simulink model "salpChain1"  (Simulink 7.8)
settings: Solver=ode15s  StartTime=0.0  StopTime=400  RelTol=1e-3
values from neighbouring files (symbols this model uses):
  evenTorque = [0 0 0]    [15RunsSmallEtta.mat]    (also in 1To10withTorque.mat = [0 0 0.2]; 1To20Nodes.mat; 1To30HeadToTail.mat; 1To35FullFlip.mat)
  N = size(INPUT,1)    [SpinCalc.m]
  oddTorque = [0 0 0]    [15RunsSmallEtta.mat]    (also in 1To10withTorque.mat = [0 0 0.2]; 1To20Nodes.mat; 1To30HeadToTail.mat; 1To35FullFlip.mat)
  sInertia = [0.0008  0  0; 0  0.0008  0; 0  0  0.0004]    [15RunsSmallEtta.mat]    (also in 1To10withTorque.mat; 1To20Nodes.mat; 1To30HeadToTail.mat; 1To35FullFlip.mat)
  sMass = 0.04    [15RunsSmallEtta.mat]    (also in 1To10withTorque.mat; 1To20Nodes.mat; 1To30HeadToTail.mat; 1To35FullFlip.mat)
  uAmplitudeEven = [-1.03766578533 1.19688881264 1.2209450799]    [15RunsSmallEtta.mat]    (also in 1To10withTorque.mat = [-0.2 0 2]; 1To20Nodes.mat = [-0.2 0 2]; 1To30HeadToTail.mat = [-0.2 0 2]; 1To35FullFlip.mat = [-0.2 0.2 2])
libraries: mblibv1 x14
settings Model: Creator=benjJohnson  LastModifiedBy=benjJohnson

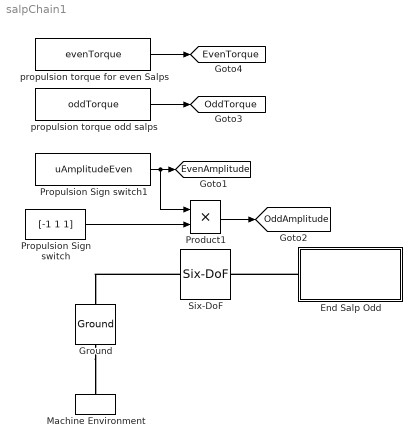
== system salpChain1 ==
  End Salp Odd : Subsystem
  Ground : mblibv1/Bodies/Ground  UpdateFromCAD=off  LeftPortType=env  RightPortType=workingframe  PhysicalDomain=Mechanical  DialogClass=GroundBlock  CoordPosition=[0 0 0]  CoordPositionUnits=m  StateVectorMgrId=-1  MachineId=[0 0]  ShowEnvPort=on
  Machine Environment : mblibv1/Bodies/Machine Environment  PortType=env  PhysicalDomain=Mechanical  DialogTemplateClass=MECH.MachineEnvironment  SyncWhenCopied=off  Gravity=[0 0 0]  GravityUnits=m/s^2  GravityAsSignal=off  Dimensionality=Auto-detect  AnalysisType=Forward dynamics  LinearAssemblyTolerance=1e-3  LinearAssemblyToleranceUnits=m  AngularAssemblyTolerance=1e-3  AngularAssemblyToleranceUnits=rad  ConstraintSolverType=Stabilizing  ConstraintRelTolerance=1e-4  ConstraintAbsTolerance=1e-4  UseRobustSingularityHandling=off  RedundancyAnalysisToleranceType=Automatically select tolerance  RedundancyAnalysisTolerance=1e-14  StatePerturbationType=Fixed  PerturbationSize=1e-5  VisualizeMachine=on  BodyVisualizationType=Use model default body geometries  BodyColorSelMode=Use model default  DefaultBodyColor=[1 0 0]
  Product1 : Product  RndMeth=Zero
  Propulsion Sign switch : Constant  Value=[-1 1 1]  VectorParams1D=off
  Propulsion Sign switch1 : Constant  Value=uAmplitudeEven  VectorParams1D=off
  Six-DoF : mblibv1/Joints/Six-DoF  LConnTagsString=__newl0  RConnTagsString=__newr0  UpdateFromCAD=off  NumSAPorts=0  CutJoint=off  MarkAsCut=off  Primitives=prismatic_prismatic  PrimitiveProps=P1$World$[1 0 0]$prismatic#P2$World$[0 1 0]$prismatic#P3$World$[0 0 1]$prismatic#S$World$[0 0 0]$spherical  DialogClass=JointBlock  P1Axis=[1 0 0]  P2Axis=[0 1 0]  P3Axis=[0 0 1]  SAxis=[0 0 0]
  propulsion torque for even Salps : Constant  Value=evenTorque  VectorParams1D=off
  propulsion torque odd salps : Constant  Value=oddTorque  VectorParams1D=off
  tag scope: EvenAmplitude=global, EvenTorque=global, OddAmplitude=global, OddTorque=global
  wires:
  Propulsion Sign switch/1 -> Product1/2
  Product1/1 -> [OddAmplitude]
  Propulsion Sign switch1/1 -> [EvenAmplitude], Product1/1
  propulsion torque for even Salps/1 -> [EvenTorque]
  propulsion torque odd salps/1 -> [OddTorque]
  connections:
  Six-DoF/LConn1 -- Ground/RConn1
  Ground/LConn1 -- Machine Environment/RConn1
  End Salp Odd/LConn1 -- Six-DoF/RConn1

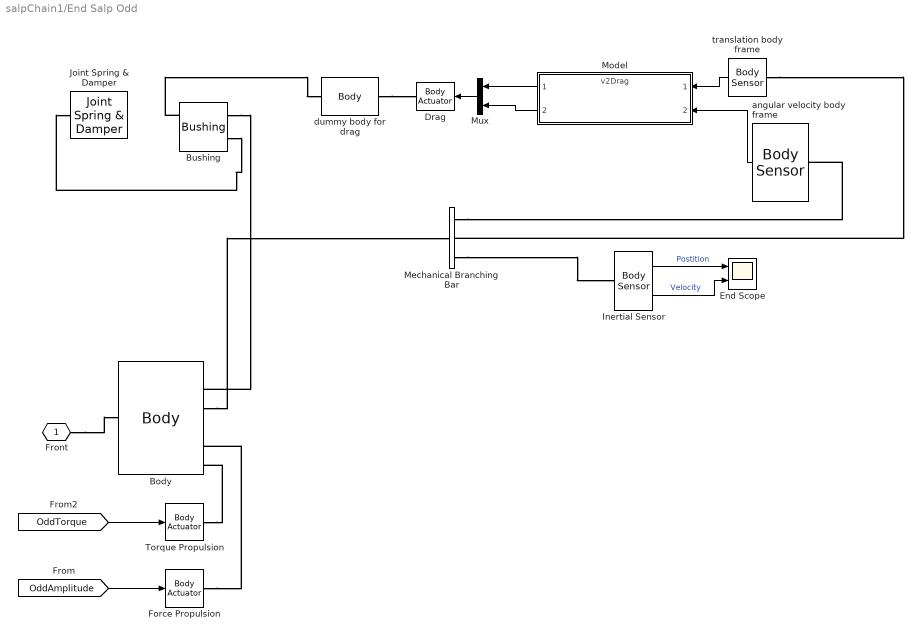
== system salpChain1/End Salp Odd ==
  Body : mblibv1/Bodies/Body  LConnTagsString=CS1  RConnTagsString=CG|CS5|CS4|CS2|CS3|CS6  UpdateFromCAD=off  DialogClass=MechanicalBodyBlock  Mass=sMass  MassUnits=kg  InertiaUnits=kg*m^2  Inertia=sInertia  Shape=Cylinder  ShapeDims=[1 1]  ShapeUnits=m  ShapeUse=false  Density=1  DensityUnits=kg/m^3  DensityUse=false  GraphicsMode=EQELLIPSE  BodyColorSelMode=COLORPALETTE  BodyColor=[0.16471 0.38431 0.27451]  AttachedToCS=CG  CG=Right$CG$frontConnect$CS1$CS1$m$[0 0 0]$Euler X-Y-Z$deg$CS1$true$none  WorkingFrames=Right$CS5$COPPosition$CG$CG$m$[0 0 0]$Euler X-Y-Z$deg$CS1$true$none#Right$CS4$[0 0 0]$CG$CG$m$[0 0 0]$Euler X-Y-Z$deg$CS1$true$none#Left$CS1$[0 0 0]$Adjoining$Adjoining$m$connectR$Euler X-Y-Z$deg$Adjoining$true$none#Right$CS2$backConnect$CG$CG$m$[0 0 0]$Euler X-Y-Z$deg$CS1$true$none#Right$CS3$propulsionPosition$CG$CG$m$[0 0 0]$Euler X-Y-Z$deg$CS1$true$none#Right$CS6$propulsionPosition$CG$CG$m$[0 0 0]$Euler X-Y-Z$deg$CS1$true$none  CGPos=frontConnect  CGRot=[0 0 0]  CS0Pos=[]  CS0Rot=[]  CS1Pos=[0 0 0]  CS1Rot=connectR  CS2Pos=backConnect  CS2Rot=[0 0 0]  CS3Pos=propulsionPosition  CS3Rot=[0 0 0]  CS4Pos=[0 0 0]  CS4Rot=[0 0 0]  CS5Pos=COPPosition  CS5Rot=[0 0 0]  CS6Pos=propulsionPosition  CS6Rot=[0 0 0]  CS7Pos=[]  CS7Rot=[]  CS8Pos=[]  CS8Rot=[]  CS9Pos=[]  CS9Rot=[]  CS10Pos=[]  CS10Rot=[]  CS11Pos=[]  CS11Rot=[]  CS12Pos=[]  CS12Rot=[]  CS13Pos=[]  CS13Rot=[]  CS14Pos=[]  CS14Rot=[]  CS15Pos=[]  CS15Rot=[]  CS16Pos=[]  CS16Rot=[]  CS17Pos=[]  CS17Rot=[]  CS18Pos=[]  CS18Rot=[]  CS19Pos=[]  CS19Rot=[]  CS20Pos=[]  CS20Rot=[]
  Bushing : mblibv1/Joints/Bushing  LConnTagsString=__newl0|SA1  RConnTagsString=__newr0|SA1  UpdateFromCAD=off  NumSAPorts=2  CutJoint=off  MarkAsCut=off  Primitives=prismatic_prismatic_prismatic  PrimitiveProps=P1$Follower$[1 0 0]$prismatic#P2$Follower$[0 1 0]$prismatic#P3$Follower$[0 0 1]$prismatic#R1$Follower$[1 0 0]$revolute#R2$Follower$[0 1 0]$revolute#R3$Follower$[0 0 1]$revolute  DialogClass=JointBlock  P1Axis=[1 0 0]  P2Axis=[0 1 0]  P3Axis=[0 0 1]  R1Axis=[1 0 0]  R2Axis=[0 1 0]  R3Axis=[0 0 1]
  Drag : mblibv1/Sensors &  Actuators/Body Actuator  UpdateFromCAD=off  PhysicalDomain=Mechanical  PortType=blob  ActuationStyle=Force  AngleUnits=deg  ArcVelocityUnits=deg/s  ArcAccelerationUnits=deg/s^2  CoordPositionUnits=m  VelocityUnits=m/s  AccelerationUnits=m/s^2  ForceUnits=N  TorqueUnits=N*m  ActiveIO=off  Width=6  DialogClass=MechanicalActuatorBlock  ReferenceFrame=Local (Body CS)  Angle=off  CoordPosition=on  Force=on  Torque=on
  End Scope : Scope  NumInputPorts=2
      settings: YMin=0~-0.1  YMax=55~0.225  SaveName=endSalp_PandV  MaxDataPoints=9000
  Force Propulsion : mblibv1/Sensors &  Actuators/Body Actuator  UpdateFromCAD=off  PhysicalDomain=Mechanical  PortType=blob  ActuationStyle=Force  AngleUnits=deg  ArcVelocityUnits=deg/s  ArcAccelerationUnits=deg/s^2  CoordPositionUnits=m  VelocityUnits=m/s  AccelerationUnits=m/s^2  ForceUnits=N  TorqueUnits=N*m  ActiveIO=off  Width=3  DialogClass=MechanicalActuatorBlock  ReferenceFrame=Local (Body CS)  Angle=off  CoordPosition=on  Force=on  Torque=off
  Inertial Sensor : mblibv1/Sensors &  Actuators/Body Sensor  UpdateFromCAD=off  PhysicalDomain=Mechanical  PortType=blob  Muxed=off  Pose=off  Angle=on  AngleUnits=deg  ArcVelocity=off  ArcVelocityUnits=deg/s  ArcAcceleration=off  ArcAccelerationUnits=deg/s^2  CoordPosition=on  CoordPositionUnits=m  Velocity=on  VelocityUnits=m/s  Acceleration=off  AccelerationUnits=m/s^2  Quaternion=on  QuaternionDT=off  QuaternionDDT=off  QuaternionUnits=off  OutputVector=[1]  ActiveIO=off  Width=6  DialogClass=MechanicalSensorBlock  ReferenceFrame=Absolute (World)
  Joint Spring & Damper : mblibv1/Force  Elements/Joint Spring & Damper  UpdateFromCAD=off  DialogClass=JointSpringDamper  JFEParameters=P1$true$kDrag(1)$bDrag(1)$0$m$m/s$N$deg$deg/s$N*m#P2$true$kDrag(2)$bDrag(2)$0$m$m/s$N$deg$deg/s$N*m#P3$true$kDrag(3)$bDrag(3)$0$m$m/s$N$deg$deg/s$N*m#R1$true$kDrag(4)$bDrag(4)$0$m$m/s$N$deg$deg/s$N*m#R2$true$kDrag(5)$bDrag(5)$0$m$m/s$N$deg$deg/s$N*m#R3$true$kDrag(6)$bDrag(6)$0$m$m/s$N$deg$deg/s$N*m#S$false$0$0$0$m$m/s$N$deg$deg/s$N*m
  Mechanical Branching Bar : mblibv1/Utilities/Mechanical Branching Bar  LConnTagsString=_newl0  RConnTagsString=__newr0|SA2|SA3  UpdateFromCAD=off  DialogClass=MechanicalBranchingBarBlock  NumSAPorts=3
  Model : ModelReference  ModelNameDialog=v2Drag  SimulationMode=Normal  ModelReferenceVersion=1.16  CopyOfModelName=v2Drag  DefaultDataLogging=on
  Mux : Mux  Inputs=2
  Torque Propulsion : mblibv1/Sensors &  Actuators/Body Actuator  UpdateFromCAD=off  PhysicalDomain=Mechanical  PortType=blob  ActuationStyle=Force  AngleUnits=deg  ArcVelocityUnits=deg/s  ArcAccelerationUnits=deg/s^2  CoordPositionUnits=m  VelocityUnits=m/s  AccelerationUnits=m/s^2  ForceUnits=N  TorqueUnits=N*m  ActiveIO=off  Width=3  DialogClass=MechanicalActuatorBlock  ReferenceFrame=Local (Body CS)  Angle=off  CoordPosition=on  Force=off  Torque=on
  angular velocity body frame : mblibv1/Sensors &  Actuators/Body Sensor  UpdateFromCAD=off  PhysicalDomain=Mechanical  PortType=blob  Muxed=off  Pose=off  Angle=on  AngleUnits=deg  ArcVelocity=on  ArcVelocityUnits=deg/s  ArcAcceleration=off  ArcAccelerationUnits=deg/s^2  CoordPosition=off  CoordPositionUnits=m  Velocity=off  VelocityUnits=m/s  Acceleration=off  AccelerationUnits=m/s^2  Quaternion=on  QuaternionDT=off  QuaternionDDT=off  QuaternionUnits=off  OutputVector=[1]  ActiveIO=off  Width=3  DialogClass=MechanicalSensorBlock  ReferenceFrame=Local (Body CS)
  dummy body for drag : mblibv1/Bodies/Body  LConnTagsString=CS1  RConnTagsString=CS2  UpdateFromCAD=off  DialogClass=MechanicalBodyBlock  Mass=sMass/100  MassUnits=kg  InertiaUnits=kg*m^2  Inertia=eye(3)/1000  Shape=Cylinder  ShapeDims=[1 1]  ShapeUnits=m  ShapeUse=false  Density=1  DensityUnits=kg/m^3  DensityUse=false  GraphicsMode=CONVHULL  BodyColorSelMode=COLORPALETTE  BodyColor=[1 0 1]  AttachedToCS=CG  CG=Left$CG$[0 0 0]$CS1$CS1$m$[0 0 0]$Euler X-Y-Z$deg$CS1$false$none  WorkingFrames=Left$CS1$[0 0 0]$Adjoining$Adjoining$m$[0 0 0]$Euler X-Y-Z$deg$Adjoining$true$none#Right$CS2$[0 0 0]$CS1$CS1$m$[0 0 0]$Euler X-Y-Z$deg$CS1$true$none  CGPos=[0 0 0]  CGRot=[0 0 0]  CS0Pos=[]  CS0Rot=[]  CS1Pos=[0 0 0]  CS1Rot=[0 0 0]  CS2Pos=[0 0 0]  CS2Rot=[0 0 0]  CS3Pos=[]  CS3Rot=[]  CS4Pos=[]  CS4Rot=[]  CS5Pos=[]  CS5Rot=[]  CS6Pos=[]  CS6Rot=[]  CS7Pos=[]  CS7Rot=[]  CS8Pos=[]  CS8Rot=[]  CS9Pos=[]  CS9Rot=[]  CS10Pos=[]  CS10Rot=[]  CS11Pos=[]  CS11Rot=[]  CS12Pos=[]  CS12Rot=[]  CS13Pos=[]  CS13Rot=[]  CS14Pos=[]  CS14Rot=[]  CS15Pos=[]  CS15Rot=[]  CS16Pos=[]  CS16Rot=[]  CS17Pos=[]  CS17Rot=[]  CS18Pos=[]  CS18Rot=[]  CS19Pos=[]  CS19Rot=[]  CS20Pos=[]  CS20Rot=[]
  translation body frame : mblibv1/Sensors &  Actuators/Body Sensor  UpdateFromCAD=off  PhysicalDomain=Mechanical  PortType=blob  Muxed=off  Pose=off  Angle=on  AngleUnits=deg  ArcVelocity=off  ArcVelocityUnits=deg/s  ArcAcceleration=off  ArcAccelerationUnits=deg/s^2  CoordPosition=off  CoordPositionUnits=m  Velocity=on  VelocityUnits=m/s  Acceleration=off  AccelerationUnits=m/s^2  Quaternion=on  QuaternionDT=off  QuaternionDDT=off  QuaternionUnits=off  OutputVector=[1]  ActiveIO=off  Width=3  DialogClass=MechanicalSensorBlock  ReferenceFrame=Local (Body CS)
  Front : PMIOPort  Port=1  Side=Left
  wires:
  translation body frame/1 -> Model/1
  Mux/1 -> Drag/1
  angular velocity body frame/1 -> Model/2
  Model/1 -> Mux/1
  Model/2 -> Mux/2
  [OddAmplitude] -> Force Propulsion/1
  [OddTorque] -> Torque Propulsion/1
  Inertial Sensor/1 -> End Scope/1  "Postition"
  Inertial Sensor/2 -> End Scope/2  "Velocity"
  connections:
  Body/RConn3 -- Mechanical Branching Bar/LConn1
  dummy body for drag/RConn1 -- Drag/RConn1
  Mechanical Branching Bar/RConn1 -- angular velocity body frame/LConn1
  translation body frame/LConn1 -- Mechanical Branching Bar/RConn2
  Bushing/RConn1 -- Body/RConn2
  Bushing/LConn1 -- dummy body for drag/LConn1
  Bushing/RConn2 -- Joint Spring & Damper/LConn1
  Front/RConn1 -- Body/LConn1
  Force Propulsion/RConn1 -- Body/RConn5
  Torque Propulsion/RConn1 -- Body/RConn6
  Mechanical Branching Bar/RConn3 -- Inertial Sensor/LConn1
